simulink model "SerialTest"  (R2020a)
settings: Solver=FixedStepAuto  StartTime=0.0  StopTime=10.0  FixedStep=1e-3  RelTol=1e-3  EnableMultiTasking=on
libraries: simulink x1, frdmk64flib x1
settings Model: ExtModeTrigDuration=5  Creator=WinnieTrandinh  LastModifiedBy=WinnieTrandinh
settings OptimizationCC: EnhancedBackFolding=on  PassReuseOutputArgsAs=Individual arguments  ZeroExternalMemoryAtStartup=off  ZeroInternalMemoryAtStartup=off  MaxStackSize=64  OptimizeBlockOrder=speed  DifferentSizesBufferReuse=on  OptimizationCustomize=off  EfficientTunableParamExpr=on
settings DebuggingCC: ParameterTunabilityLossMsg=error
settings HardwareCC: ProdBitPerPointer=32  ProdBitPerSizeT=32  ProdBitPerPtrDiffT=32  ProdLargestAtomicInteger=Long  ProdLargestAtomicFloat=Double  ProdWordSize=32  ProdHWDeviceType=ARM Compatible->ARM Cortex
settings SFSimCC: MATLABDynamicMemAlloc=off
settings RTWCC: SystemTargetFile=ert.tlc  HardwareBoard=NXP FRDM-K64F  TemplateMakefile=ert_default_tmf  Toolchain=GNU Tools for ARM Embedded Processors
settings CodeAppCC: ForceParamTrailComments=on  IgnoreCustomStorageClasses=off  OperatorAnnotations=on  SimulinkDataObjDesc=on  SFDataObjDesc=on  InsertBlockDesc=on

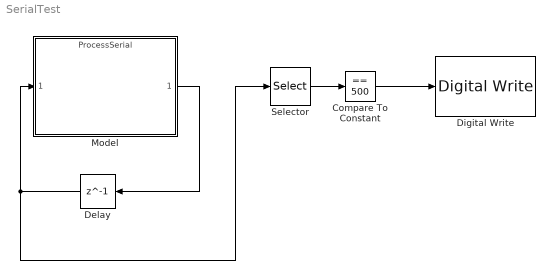
== system SerialTest ==
  Compare To Constant : simulink/Logic and Bit Operations/Compare To Constant  relop===  const=500  OutDataTypeStr=boolean
  Delay : Delay  DelayLength=1  InitialCondition=[1000 5 10 5 10 300 400 3.5 3.5 50 0.1 16 5000 5000 1 100 1 1 1]
  Digital Write : frdmk64flib/Digital Write  Whichpin=RED_LED
  Model : ModelReference  ModelNameDialog=ProcessSerial.slx  SimulationMode=Normal  ModelReferenceVersion=1.7
  Selector : Selector  IndexOptions=Index vector (dialog)  Indices=[7]  OutputSizes=1
  wires:
  Model/1 -> Delay/1
  Delay/1 -> Model/1, Selector/1
  Selector/1 -> Compare To Constant/1
  Compare To Constant/1 -> Digital Write/1
